simulink model "EngCylTest"  (Simulink 8.1)
settings: Solver=ode4  StartTime=0.0  StopTime=10  FixedStep=1e-3  RelTol=1e-3
values from neighbouring files (symbols this model uses):
  B = [B1;B2]    [GensetRespOptimiztion.m]    (also in GensetRespOptimiztionTorstein.m; Init8RTFLEX68D.m = 0.68; init_MVM.m = 0.127)
  stroke = 2.72    [Init8RTFLEX68D.m]
libraries: EngineSysteSubmodel x1
settings Model: Creator=yum  LastModifiedBy=yum
settings DataIOCC: SignalLoggingSaveFormat=Dataset  InspectSignalLogs=on  ReturnWorkspaceOutputs=on
settings OptimizationCC: ExpressionDepthLimit=128
settings DebuggingCC: FcnCallInpInsideContextMsg=EnableAllAsError
settings GRTTargetCC: CombineOutputUpdateFcns=on  GRTInterface=off

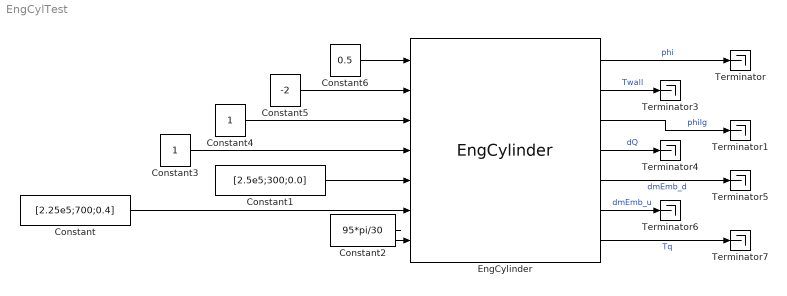
== system EngCylTest ==
  Constant : Constant  Value=[2.25e5;700;0.4]
  Constant1 : Constant  Value=[2.5e5;300;0.0]
  Constant2 : Constant  Value=95*pi/30
  Constant3 : Constant
  Constant4 : Constant
  Constant5 : Constant  Value=-2
  Constant6 : Constant  Value=0.5
  EngCylinder : EngineSysteSubmodel/EngCylinder  fs=fs  nStroke=nStroke  hn=hn  nCyl=nCyl  iCyl=1  B=B  stroke=stroke  lambdaCrank=lambdaCrank  aCrank=stroke/2  X=X  Y=Y  r=r  nPort=nPort  liftMax=liftMax  Dv=Dv  beta=beta  w=w  Dp=Dp  Ds=Ds  cAVVUpRef=cAVVUpRef  cAVVDownRef=cAVVDownRef  liftUpRef=liftUpRef  liftDownRef=liftDownRef  cAStartRef=cAStartRef  dCALiftUp=dCALiftUp  dCALiftDown=dCALiftDown  dCALiftTopRef=dCALiftTopRef  mCp=mCp  cCylHT=cCylHT  cAlpha=cAlpha  mqfCycMax=mqfCycMax  wiebePara=wiebePara  phi0=phi0  m0=mCyl0  E0=ECyl0  mb0=mbCyl0  V0=vCyl0  phi0A=phi0rad  m0A=mCyl0  E0A=ECyl0  mb0A=mbCyl0  V0A=vCyl0
  Terminator{,1,3..7} (7 alike) : Terminator
  wires:
  Constant/1 -> EngCylinder/6
  Constant1/1 -> EngCylinder/5
  Constant2/1 -> EngCylinder/7
  Constant3/1 -> EngCylinder/4
  Constant4/1 -> EngCylinder/3
  Constant5/1 -> EngCylinder/2
  Constant6/1 -> EngCylinder/1
  EngCylinder/1 -> Terminator/1  "phi"
  EngCylinder/3 -> Terminator1/1  "phiIg"
  EngCylinder/2 -> Terminator3/1  "Twall"
  EngCylinder/4 -> Terminator4/1  "dQ"
  EngCylinder/5 -> Terminator5/1  "dmEmb_d"
  EngCylinder/6 -> Terminator6/1  "dmEmb_u"
  EngCylinder/7 -> Terminator7/1  "Tq"
